simulink model "BKYB_zadanie2_PD_Berg_sim_21a"  (R2021a)
settings: Solver=VariableStepAuto  StartTime=0.0  StopTime=600  RelTol=1e-3
values from neighbouring files (symbols this model uses):
  Ib = 6.5    [params.m]
  p2 = Pop(i,1)    [fitness_dk.m]    (also in params.m = best_ch(1,end))
undefined symbols (not defined in the file or in its folder): G0, KI, S1b, S2b, sampleTime, SI, TI, vb, VG, VI
settings Model: Creator=Jurko  LastModifiedBy=DFUNDO
settings DebuggingCC: UnconnectedInputMsg=none  UnconnectedOutputMsg=none  UnconnectedLineMsg=none
settings ModelReferenceCC: EnableRefExpFcnMdlSchedulingChecks=off
settings RTWCC: Description=Generic Real-Time Target  DLArmComputeVersion=20.02.1

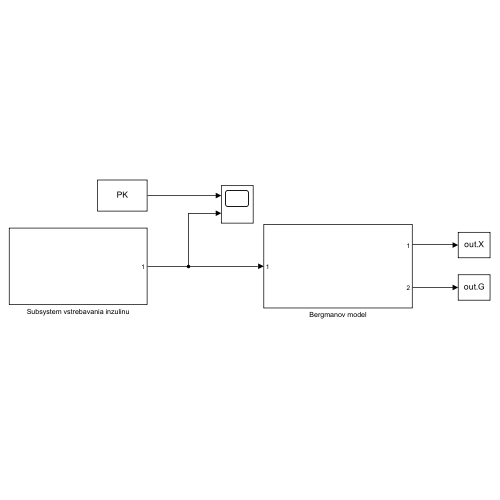
[thumbnail: Simulink's stored preview of the top-level diagram]
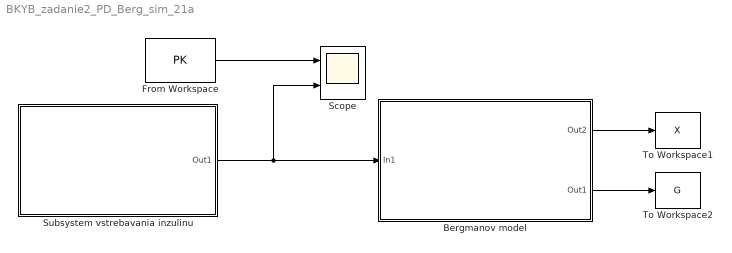
== system BKYB_zadanie2_PD_Berg_sim_21a ==
  Bergmanov model : Subsystem
  From Workspace : FromWorkspace  VariableName=PK
  Scope : Scope  NumInputPorts=2
  Subsystem vstrebavania inzulinu : Subsystem
  To Workspace1 : ToWorkspace  VariableName=X  SampleTime=sampleTime
  To Workspace2 : ToWorkspace  VariableName=G  SampleTime=sampleTime
  wires:
  Subsystem vstrebavania inzulinu/1(Out1) -> Bergmanov model/1(In1), Scope/2
  From Workspace/1 -> Scope/1
  Bergmanov model/1(Out2) -> To Workspace1/1
  Bergmanov model/2(Out1) -> To Workspace2/1

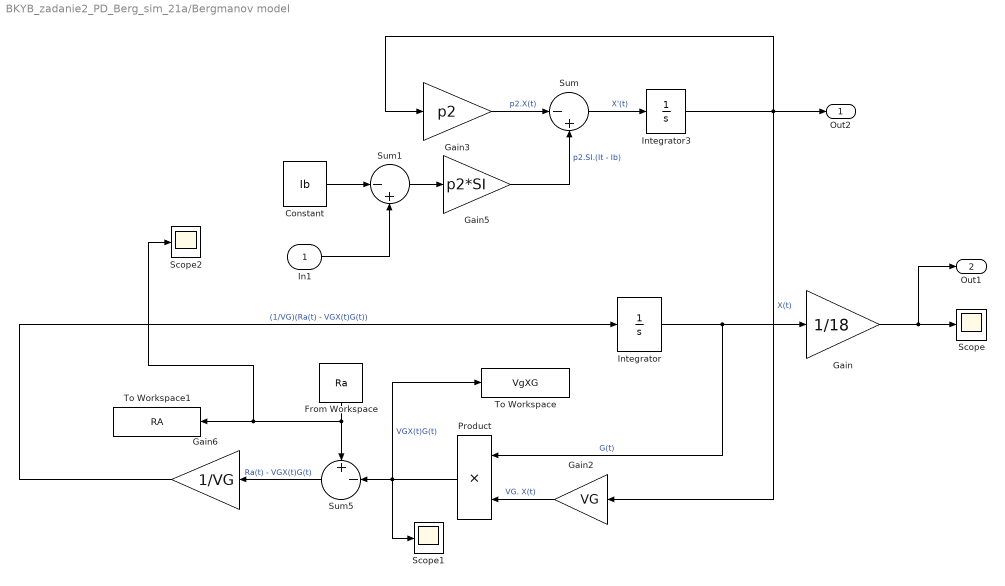
== system BKYB_zadanie2_PD_Berg_sim_21a/Bergmanov model ==
  In1 : Inport
  Constant : Constant  Value=Ib
  From Workspace : FromWorkspace  VariableName=Ra  OutDataTypeStr=double
  Gain : Gain  Gain=1/18
  Gain2 : Gain  Gain=VG
  Gain3 : Gain  Gain=p2
  Gain5 : Gain  Gain=p2*SI
  Gain6 : Gain  Gain=1/VG
  Integrator : Integrator  InitialCondition=G0
  Integrator3 : Integrator
  Product : Product
  Scope : Scope
  Scope1 : Scope
  Scope2 : Scope
  Sum : Sum  Inputs=|-+
  Sum1 : Sum  Inputs=|-+
  Sum5 : Sum  Inputs=+-|
  To Workspace : ToWorkspace  VariableName=VgXG  SampleTime=sampleTime
  To Workspace1 : ToWorkspace  VariableName=RA  SampleTime=sampleTime
  Out2 : Outport
  Out1 : Outport  Port=2
  wires:
  In1/1 -> Sum1/2
  Gain3/1 -> Sum/1  "p2.X(t)"
  Sum1/1 -> Gain5/1
  Sum/1 -> Integrator3/1  "X'(t)"
  Constant/1 -> Sum1/1
  Integrator3/1 -> Gain2/1, Out2/1, Gain3/1  "X(t)"
  Gain5/1 -> Sum/2  "p2.SI.(It - Ib)"
  Integrator/1 -> Gain/1, Product/1  "G(t)"
  From Workspace/1 -> Sum5/1, Scope2/1, To Workspace1/1
  Gain2/1 -> Product/2  "VG. X(t)"
  Gain6/1 -> Integrator/1  "(1/VG)(Ra(t) - VGX(t)G(t))"
  Sum5/1 -> Gain6/1  "Ra(t) - VGX(t)G(t)"
  Product/1 -> To Workspace/1, Scope1/1, Sum5/2  "VGX(t)G(t)"
  Gain/1 -> Out1/1, Scope/1

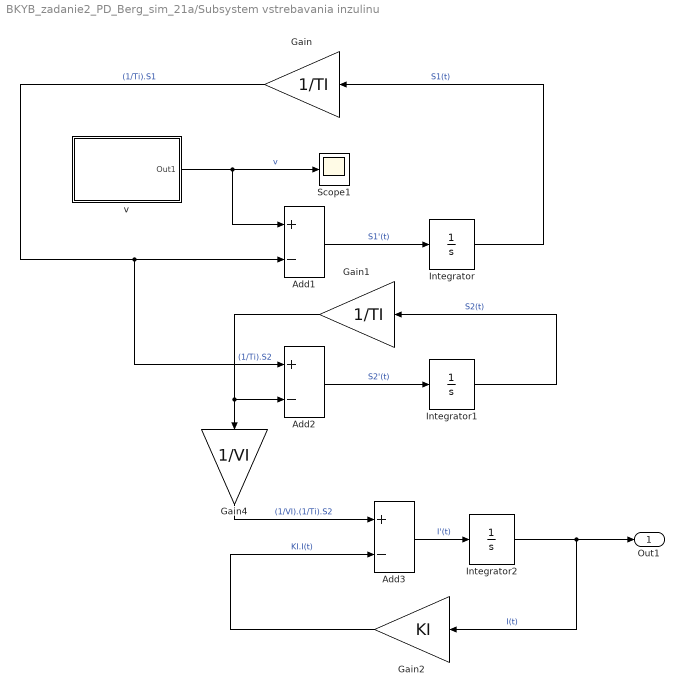
== system BKYB_zadanie2_PD_Berg_sim_21a/Subsystem vstrebavania inzulinu ==
  Add1 : Sum  Inputs=+-
  Add2 : Sum  Inputs=+-
  Add3 : Sum  Inputs=+-
  Gain : Gain  Gain=1/TI
  Gain1 : Gain  Gain=1/TI
  Gain2 : Gain  Gain=KI
  Gain4 : Gain  Gain=1/VI
  Integrator : Integrator  InitialCondition=S1b
  Integrator1 : Integrator  InitialCondition=S2b
  Integrator2 : Integrator  InitialCondition=Ib
  Scope1 : Scope
  v : Subsystem
  Out1 : Outport
  wires:
  Gain4/1 -> Add3/1  "(1/VI).(1/Ti).S2"
  Gain2/1 -> Add3/2  "KI.I(t)"
  Add3/1 -> Integrator2/1  "I'(t)"
  Gain/1 -> Add1/2, Add2/1  "(1/Ti).S1"
  Integrator2/1 -> Out1/1, Gain2/1  "I(t)"
  Integrator1/1 -> Gain1/1  "S2(t)"
  Gain1/1 -> Gain4/1, Add2/2  "(1/Ti).S2"
  v/1(Out1) -> Scope1/1, Add1/1  "v"
  Add2/1 -> Integrator1/1  "S2'(t)"
  Add1/1 -> Integrator/1  "S1'(t)"
  Integrator/1 -> Gain/1  "S1(t)"

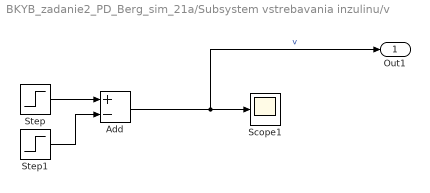
== system BKYB_zadanie2_PD_Berg_sim_21a/Subsystem vstrebavania inzulinu/v ==
  Add : Sum  Inputs=+-
  Scope1 : Scope
  Step : Step  Time=0  After=vb + 40000  SampleTime=0
  Step1 : Step  Time=5  After=40000  SampleTime=0
  Out1 : Outport
  wires:
  Step/1 -> Add/1
  Add/1 -> Out1/1, Scope1/1  "v"
  Step1/1 -> Add/2
